simulink model "simulink_aufg1_a"  (Simulink 7.7)
settings: Solver=ode45  StartTime=0.0  StopTime=10.0  RelTol=1e-3
libraries: simulink x2
settings Model: Creator=myers  LastModifiedBy=myers

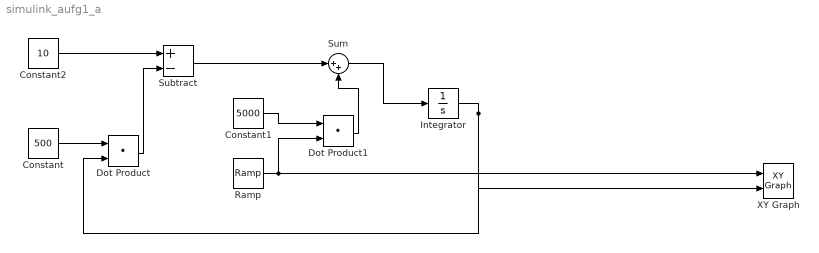
== system simulink_aufg1_a ==
  Constant : Constant  Value=500
  Constant1 : Constant  Value=5000
  Constant2 : Constant  Value=10
  Dot Product : DotProduct  InputSameDT=on  OutDataTypeStr=Inherit: Inherit via internal rule
  Dot Product1 : DotProduct  InputSameDT=on  OutDataTypeStr=Inherit: Inherit via internal rule
  Integrator : Integrator  InitialCondition=1
  Ramp : simulink/Sources/Ramp  SystemSampleTime=-1  slope=1  start=0  X0=0
  Subtract : Sum  Inputs=+-
  Sum : Sum  Inputs=|++
  XY Graph : simulink/Sinks/XY Graph  SystemSampleTime=-1  xmin=0  xmax=0.3  ymin=0  ymax=2.5  st=-1
  wires:
  Constant/1 -> Dot Product/1
  Constant2/1 -> Subtract/1
  Dot Product/1 -> Subtract/2
  Subtract/1 -> Sum/1
  Constant1/1 -> Dot Product1/1
  Sum/1 -> Integrator/1
  Integrator/1 -> Dot Product/2, XY Graph/2
  Ramp/1 -> Dot Product1/2, XY Graph/1
  Dot Product1/1 -> Sum/2
